simulink model "P1_linear_models_simplified"  (Simulink 7.9)
settings: Solver=ode45  StartTime=0.0  StopTime=10.0  RelTol=1e-3
undefined symbols (not defined in the file): h_high_cm, h_low_cm, h_mid_cm, k1_high, k1_low, k1_mid, k2_high, k2_low, k2_mid, u_high, u_low, u_mid
settings Model: Creator=matias  LastModifiedBy=matias

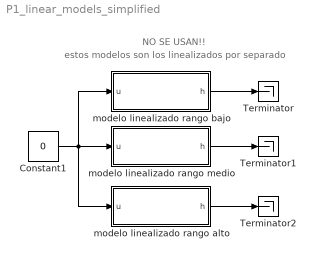
== system P1_linear_models_simplified ==
  note: estos modelos son los linealizados por separado
  note: NO SE USAN!!
  Constant1 : Constant  Value=0
  Terminator : Terminator
  Terminator1 : Terminator
  Terminator2 : Terminator
  modelo linealizado rango alto : Subsystem
  modelo linealizado rango bajo : Subsystem
  modelo linealizado rango medio : Subsystem
  wires:
  modelo linealizado rango bajo/1(h) -> Terminator/1
  modelo linealizado rango medio/1(h) -> Terminator1/1
  modelo linealizado rango alto/1(h) -> Terminator2/1
  Constant1/1 -> modelo linealizado rango medio/1(u), modelo linealizado rango bajo/1(u), modelo linealizado rango alto/1(u)

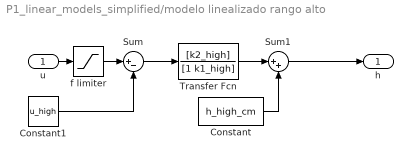
== system P1_linear_models_simplified/modelo linealizado rango alto ==
  u : Inport
  Constant : Constant  Value=h_high_cm
  Constant1 : Constant  Value=u_high
  Sum : Sum  Inputs=|+-
  Sum1 : Sum  Inputs=|++
  Transfer Fcn : TransferFcn  Numerator=[k2_high]  Denominator=[1 k1_high]
  f limiter : Saturate  UpperLimit=100  LowerLimit=0
  h : Outport
  wires:
  Constant1/1 -> Sum/2
  Sum1/1 -> h/1
  Constant/1 -> Sum1/2
  f limiter/1 -> Sum/1
  u/1 -> f limiter/1
  Sum/1 -> Transfer Fcn/1
  Transfer Fcn/1 -> Sum1/1

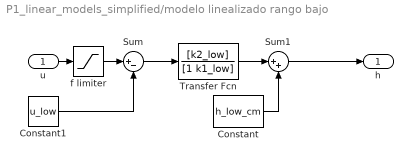
== system P1_linear_models_simplified/modelo linealizado rango bajo ==
  u : Inport
  Constant : Constant  Value=h_low_cm
  Constant1 : Constant  Value=u_low
  Sum : Sum  Inputs=|+-
  Sum1 : Sum  Inputs=|++
  Transfer Fcn : TransferFcn  Numerator=[k2_low]  Denominator=[1 k1_low]
  f limiter : Saturate  UpperLimit=100  LowerLimit=0
  h : Outport
  wires:
  Constant1/1 -> Sum/2
  Sum1/1 -> h/1
  Constant/1 -> Sum1/2
  f limiter/1 -> Sum/1
  u/1 -> f limiter/1
  Sum/1 -> Transfer Fcn/1
  Transfer Fcn/1 -> Sum1/1

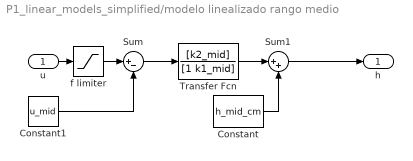
== system P1_linear_models_simplified/modelo linealizado rango medio ==
  u : Inport
  Constant : Constant  Value=h_mid_cm
  Constant1 : Constant  Value=u_mid
  Sum : Sum  Inputs=|+-
  Sum1 : Sum  Inputs=|++
  Transfer Fcn : TransferFcn  Numerator=[k2_mid]  Denominator=[1 k1_mid]
  f limiter : Saturate  UpperLimit=100  LowerLimit=0
  h : Outport
  wires:
  Constant1/1 -> Sum/2
  Sum1/1 -> h/1
  Constant/1 -> Sum1/2
  f limiter/1 -> Sum/1
  u/1 -> f limiter/1
  Sum/1 -> Transfer Fcn/1
  Transfer Fcn/1 -> Sum1/1
